simulink model "untitled"  (R2016a)
settings: Solver=VariableStepAuto  StartTime=0.0  StopTime=inf  RelTol=1e-3
undefined symbols (not defined in the file or in its folder): Pose
libraries: robotlib x3
settings Model: Creator=Administrator  LastModifiedBy=Administrator

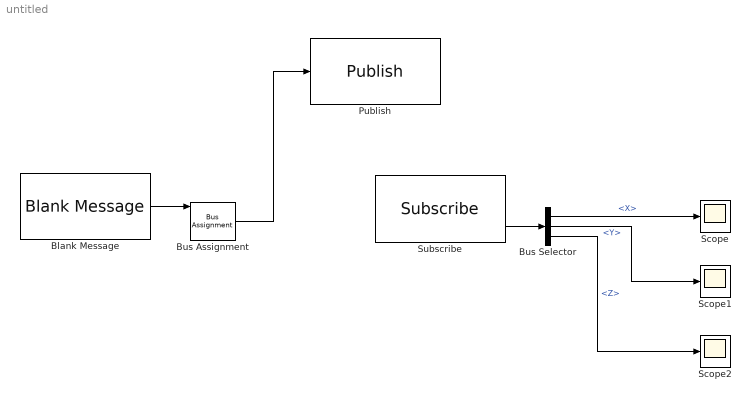
== system untitled ==
  Blank Message : robotlib/Blank Message  SourceLibraryInfo=This block requires Robotics System Toolbox  messageType=geometry_msgs/PoseStamped  SampleTime=inf
  Bus Assignment : BusAssignment  AssignedSignals=Pose.Position.X,Pose.Position.Y,Pose.Position.Z
  Bus Selector : BusSelector  OutputSignals=Pose.Position.X,Pose.Position.Y,Pose.Position.Z
  Publish : robotlib/Publish  SourceLibraryInfo=This block requires Robotics System Toolbox  topicSource=Specify your own  topic=/matlab_msgs  messageType=geometry_msgs/PoseStamped  messageQueueLength=1
  Scope : Scope
  Scope1 : Scope
  Scope2 : Scope
  Subscribe : robotlib/Subscribe  SourceLibraryInfo=This block requires Robotics System Toolbox  topicSource=Select from ROS network  topic=/uav1/mavros/local_position/pose  messageType=geometry_msgs/PoseStamped  sampleTime=-1  messageQueueLength=1
  wires:
  Subscribe/2 -> Bus Selector/1
  Bus Selector/1 -> Scope/1  "<X>"
  Bus Selector/2 -> Scope1/1  "<Y>"
  Bus Selector/3 -> Scope2/1  "<Z>"
  Blank Message/1 -> Bus Assignment/1
  Bus Assignment/1 -> Publish/1
